simulink model "prism_pprc_average_tb"  (R2024b)
settings: Solver=ode4  StartTime=0.0  StopTime=.0025  FixedStep=1e-7  RelTol=1e-3
settings Model: Creator=hj000  LastModifiedBy=hj000

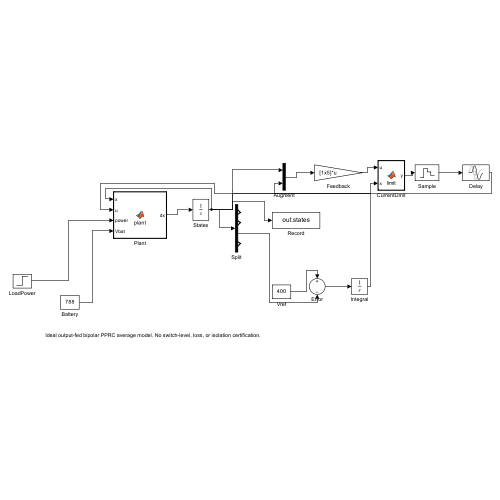
[thumbnail: Simulink's stored preview of the top-level diagram]
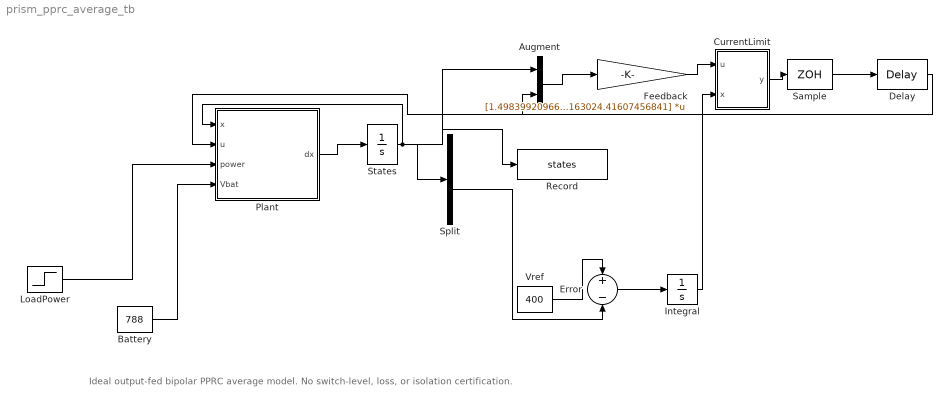
== system prism_pprc_average_tb ==
  note: Ideal output-fed bipolar PPRC average model. No switch-level, loss, or isolation certification.
  Augment : Mux  Inputs=2
  Battery : Constant  Value=788
  CurrentLimit : MATLAB Function  TreatAsAtomicUnit=on
  Delay : TransportDelay  DelayTime=5e-6  InitialOutput=12.695755342865944
  Error : Sum  Inputs=+-
  Feedback : Gain  Gain=[1.4983992096641778 -14.815248455652227 -4.0069620337297245 -1.5433537330744096 163024.41607456841]  Multiplication=Matrix(K*u)
  Integral : Integrator  InitialCondition=0.010473434780339764
  LoadPower : Step  Time=.001  Before=5000  After=29000  SampleTime=0
  Plant : MATLAB Function  TreatAsAtomicUnit=on
  Record : ToWorkspace  VariableName=states  SaveFormat=Timeseries  SampleTime=-1
  Sample : ZeroOrderHold  SampleTime=5e-6
  Split : Demux
  States : Integrator  InitialCondition=[12.695755342865944;6.1675839705258308;400;12.695755342865944]
  Vref : Constant  Value=400
  wires:
  Plant/1(dx) -> States/1
  States/1 -> Plant/1(x), Split/1, Augment/1, CurrentLimit/2(x), Record/1
  Delay/1 -> Plant/2(u)
  LoadPower/1 -> Plant/3(power)
  Battery/1 -> Plant/4(Vbat)
  Integral/1 -> Augment/2
  Augment/1 -> Feedback/1
  Feedback/1 -> CurrentLimit/1(u)
  CurrentLimit/1(y) -> Sample/1
  Sample/1 -> Delay/1
  Vref/1 -> Error/1
  Split/3 -> Error/2
  Error/1 -> Integral/1

== matlab function prism_pprc_average_tb/CurrentLimit ==
  data: u input; y output; x input
function y=limit(u,x)
cap=min([80.0800800800801,80.0800800800801*max(x(3),0)/400,8000/max(abs(x(2)),1e-9)]);
y=min(cap,max(-cap,u));
end

== matlab function prism_pprc_average_tb/Plant ==
  data: x input; u input; dx output; power input; Vbat input
function dx=plant(x,u,power,Vbat)
ip=x(1); vs=x(2); vb=x(3); id=x(4);
dx=[(Vbat/2-.0132*ip+vs-vb)/1.5e-6; (id-ip)/100e-6; (ip-(power+vs*id)/vb)/400e-6; (u-id)/1e-5];
end
